simulink model "recreere_sim"  (R2024a)
settings: Solver=VariableStepAuto  StartTime=0.0  StopTime=400  RelTol=1e-3
libraries: fod x4
settings Model: Creator=bistr  LastModifiedBy=bistr

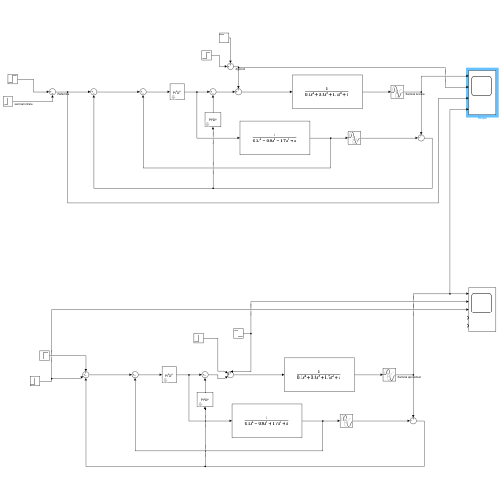
[thumbnail: Simulink's stored preview of the top-level diagram]
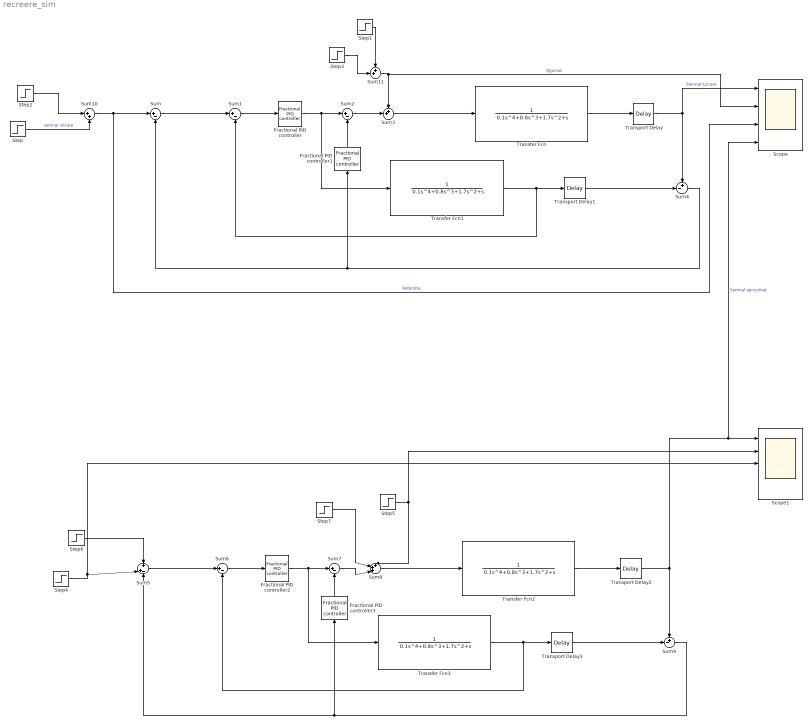
== system recreere_sim ==
  Fractional PID controller : fod/Fractional PID controller  Kp=0  Ki=0.1263  lambda=0.1218  Kd=0.2238  mic=0.8782  freqRange=[0.0000001, 1000000]  N=10
      settings: SourceProductName=FOMCON Toolbox
  Fractional PID controller1 : fod/Fractional PID controller  Kp=0  Ki=0.1263  lambda=0.1218  Kd=0.2238  mic=0.8782  freqRange=[0.001, 1000]  N=5
      settings: SourceProductName=FOMCON Toolbox
  Fractional PID controller2 : fod/Fractional PID controller  Kp=0  Ki=0.072507  lambda=0.31221  Kd=0.021901  mic=1-0.31221  freqRange=[0.1, 1000]  N=10
      settings: SourceProductName=FOMCON Toolbox
  Fractional PID controller3 : fod/Fractional PID controller  Kp=0  Ki=0.072507  lambda=0.31221  Kd=0.021901  mic=1-0.31221  freqRange=[0.1, 1000]  N=10
      settings: SourceProductName=FOMCON Toolbox
  Scope : Scope  NumInputPorts=4
  Scope1 : Scope  NumInputPorts=5
  Step : Step  Time=0  SampleTime=0
  Step1 : Step  Time=100  After=-0.1  SampleTime=0
  Step2 : Step  Time=200  SampleTime=0
  Step3 : Step  Time=300  After=0.1  SampleTime=0
  Step4 : Step  Time=0  SampleTime=0
  Step5 : Step  Time=100  After=-0.1  SampleTime=0
  Step6 : Step  Time=200  SampleTime=0
  Step7 : Step  Time=300  After=0.1  SampleTime=0
  Sum{,1..2,6..7} (5 alike) : Sum  Inputs=|+-
  Sum10 : Sum  Inputs=|++
  Sum11 : Sum  Inputs=++|
  Sum3 : Sum  Inputs=++|
  Sum4 : Sum  Inputs=+-|
  Sum5 : Sum  Inputs=+|+-
  Sum8 : Sum  Inputs=+++|
  Sum9 : Sum  Inputs=+-|
  Transfer Fcn{,1..3} (4 alike) : TransferFcn  Denominator="[0.1  0.8  1.7  1 0]"
  Transport Delay{,1..3} (4 alike) : TransportDelay  DelayTime=2
  wires:
  Sum/1 -> Sum1/1
  Sum1/1 -> Fractional PID controller/1
  Fractional PID controller/1 -> Transfer Fcn1/1, Sum2/1
  Sum2/1 -> Sum3/2
  Sum3/1 -> Transfer Fcn/1
  Transfer Fcn/1 -> Transport Delay/1
  Transport Delay/1 -> Sum4/1, Scope/1  "Semnal lucrare"
  Transfer Fcn1/1 -> Sum1/2, Transport Delay1/1
  Transport Delay1/1 -> Sum4/2
  Sum4/1 -> Sum/2, Fractional PID controller1/1
  Fractional PID controller1/1 -> Sum2/2
  Step4/1 -> Sum5/2, Scope1/3
  Fractional PID controller3/1 -> Sum7/2
  Transport Delay3/1 -> Sum9/2
  Transfer Fcn3/1 -> Sum6/2, Transport Delay3/1
  Sum9/1 -> Fractional PID controller3/1, Sum5/3
  Step7/1 -> Sum8/2
  Step6/1 -> Sum5/1
  Sum8/1 -> Transfer Fcn2/1
  Transport Delay2/1 -> Sum9/1, Scope/4, Scope1/1  "Semnal aproximat"
  Transfer Fcn2/1 -> Transport Delay2/1
  Sum7/1 -> Sum8/3
  Fractional PID controller2/1 -> Transfer Fcn3/1, Sum7/1
  Sum6/1 -> Fractional PID controller2/1
  Sum5/1 -> Sum6/1
  Step5/1 -> Sum8/1, Scope1/2
  Step2/1 -> Sum10/1
  Step/1 -> Sum10/2  "semnal intrare"
  Sum10/1 -> Sum/1, Scope/3  "Referinta"
  Step3/1 -> Sum11/2
  Sum11/1 -> Sum3/1, Scope/2  "Zgomot"
  Step1/1 -> Sum11/1
